simulink model "Untitled"  (R2016b)
settings: Solver=VariableStepAuto  StartTime=0.0  StopTime=10.0  RelTol=1e-3
undefined symbols (not defined in the file): designMultirateFIR
libraries: dspsnks4 x1, dspmlti4 x1, dspvision x1
settings Model: Creator=ssa  LastModifiedBy=ssa

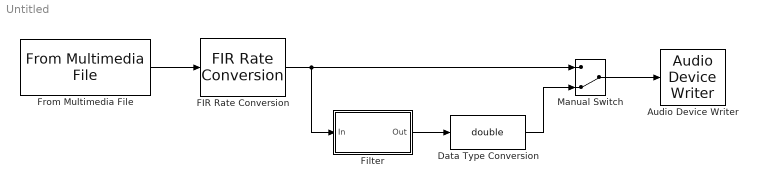
== system Untitled ==
  Audio Device Writer : dspsnks4/Audio Device Writer  Driver=DirectSound  Device=Default  InheritSampleRate=on  SampleRate=44100  BitDepth=16-bit integer  BufferSize=4096  NumBuffers=10  DefaultOutputChannelMapping=on  OutputChannelMapping=1:2  OutputNumUnderrunSamples=off  DriverIdx=1  DeviceWarnFlag=''
  Data Type Conversion : DataTypeConversion  OutDataTypeStr=double
  FIR Rate Conversion : dspmlti4/FIR Rate Conversion  FilterSource=Auto  L=160  h=designMultirateFIR(3,2)  M=147  FilterObject=FRC  roundingMode=Floor  overflowMode=off  firstCoeffDataTypeStr=Inherit: Same word length as input  firstCoeffMin=[]  firstCoeffMax=[]  firstCoeffLastDataTypeStr=Inherit: Same word length as input  outputDataTypeStr=Inherit: Same as accumulator  outputMin=[]  outputMax=[]  outputLastDataTypeStr=Inherit: Same as accumulator
  Filter : Subsystem  Tag=BlockMethodSubSystem
  From Multimedia File : dspvision/From Multimedia File  inputFilename=C:\Users\ssa\Desktop\input.wav  loop=on  numPlays=inf  outputStreams=Audio only  videoDataType=single  audioDataType=double  inheritSampleTime=on  userDefinedSampleTime=1/30  noAudioOutput=off  isIntensityVideo=off  fourcc=RGB  colorVideoFormat=Separate color signals  outputEOF=off  dataOrg=Column-major  audioFrameSize=1470  computeAudioFrameSize=off  outSamplingMode=Sample based
  Manual Switch : ManualSwitch  CurrentSetting=0
  wires:
  Filter/1(Out) -> Data Type Conversion/1
  FIR Rate Conversion/1 -> Filter/1(In), Manual Switch/1
  From Multimedia File/1 -> FIR Rate Conversion/1
  Data Type Conversion/1 -> Manual Switch/2
  Manual Switch/1 -> Audio Device Writer/1

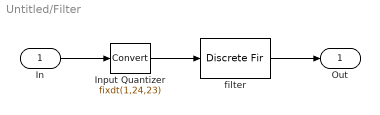
== system Untitled/Filter ==
  In : Inport
  Input Quantizer : DataTypeConversion  OutDataTypeStr=fixdt(1,24,23)  RndMeth=Round  SaturateOnIntegerOverflow=on
  filter : DiscreteFir  Coefficients=[-0.001997700337373762 -0.0050522246581640434 -0.0083320491229777194 -0.010538850721420936 -0.0092860536915670387 -0.0046562663643371152 0.0021277174805205234 0.0072199961677809352 0.007809197157319165 0.0027555956690001422 -0.0048457250469423991 -0.010213208867295952 -0.0088139437322014326 -0.00069035217320588321 0.0096039776561191014 0.014631329212397702 0.009736841326927528 -0.003618876094369877 -0.017051301049571504 -0.020554496157747987 -0.0090655570931518249 0.012214391051198006 0.029644835179847843 0.028713128973647292 0.0046994479084188938 -0.031500546980885467 -0.056127791025032278 -0.044636269121911668 0.013765567207902665 0.10696735093216615 0.20287290240459227 0.26350256726308308 0.26350256726308308 0.20287290240459227 0.10696735093216615 0.013765567207902665 -0.044636269121911668 -0.056127791025032278 -0.031500546980885467 0.0046994479084188938 0.028713128973647292 0.029644835179847843 0.012214391051198006 -0.0090655570931518249 -0.020554496157747987 -0.017051301049571504 -0.003618876094369877 0.009736841326927528 0.014631329212397702 0.0096039776561191014 -0.00069035217320588321 -0.0088139437322014326 -0.010213208867295952 -0.0048457250469423991 0.0027555956690001422 0.007809197157319165 0.0072199961677809352 0.0021277174805205234 -0.0046562663643371152 -0.0092860536915670387 -0.010538850721420936 -0.0083320491229777194 -0.0050522246581640434 -0.001997700337373762]  InputProcessing=Columns as channels (frame based)  CoefDataTypeStr=fixdt(true,16,16)  ProductDataTypeStr=fixdt(true,31,31)  AccumDataTypeStr=fixdt(true,34,31)  OutDataTypeStr=fixdt(true,32,30)  RndMeth=Convergent
  Out : Outport
  wires:
  In/1 -> Input Quantizer/1
  Input Quantizer/1 -> filter/1
  filter/1 -> Out/1
